simulink model "Q2_W3"  (R2020b)
settings: Solver=VariableStepAuto  StartTime=0.0  StopTime=10.0  RelTol=1e-3
settings Model: EnablePacing=on  Creator=hp  LastModifiedBy=hp

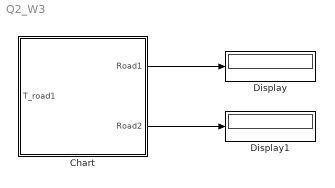
== system Q2_W3 ==
  Chart : Stateflow chart  TreatAsAtomicUnit=on
  Display : Display
  Display1 : Display
  wires:
  Chart/1(Road1) -> Display/1
  Chart/2(Road2) -> Display1/1

== stateflow chart Q2_W3/Chart ==
  state RedGreen
    entry:
    Road1=1;
    Road2=3;
  state RedYellow
    entry:
    Road1=1;
    Road2=2;
  state RedGreenIntermediate
    entry:
    Road1=1;
    Road2=3;
  state YellowRed
    entry:
    Road1=2;
    Road2=1;
  state ?
  state GreenRed
  (default) -> RedGreen : {delay=40;}
  RedGreen -> RedGreen [order 1] : [delay>0]{delay=delay-1;}
  RedYellow -> RedYellow [order 1] : [delay>0]{delay=delay-1;}
  RedGreenIntermediate -> RedYellow : [T_road1==1]{delay=20}
  RedGreen -> RedGreenIntermediate [order 2] : [delay==0]
  RedYellow -> YellowRed [order 2] : [delay==0]{delay=10;}
  YellowRed -> YellowRed [order 1] : [delay>0]{delay=delay-1;}
  YellowRed -> GreenRed [order 2] : [delay==0]{delay=40}
  GreenRed -> GreenRed : [delay>0]{delay=delay-1;}
  data: delay local; Road1 output; Road2 output; T_road1 input
